simulink model "demodulation"  (R2022b)
settings: Solver=VariableStepAuto  StartTime=0.0  StopTime=1  RelTol=1e-3
libraries: commsynccomp2 x2, dspfdesign x1
settings Model: Creator=Samin  LastModifiedBy=Samin

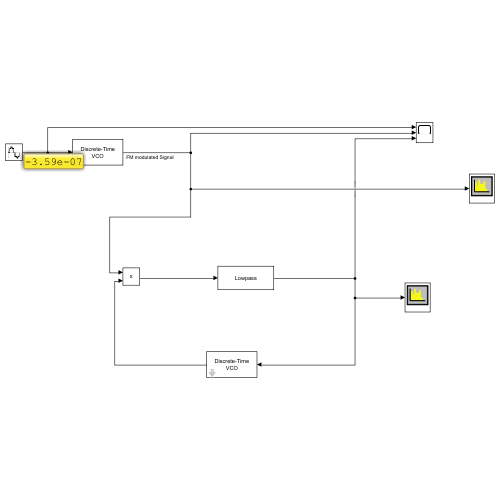
[thumbnail: Simulink's stored preview of the top-level diagram]
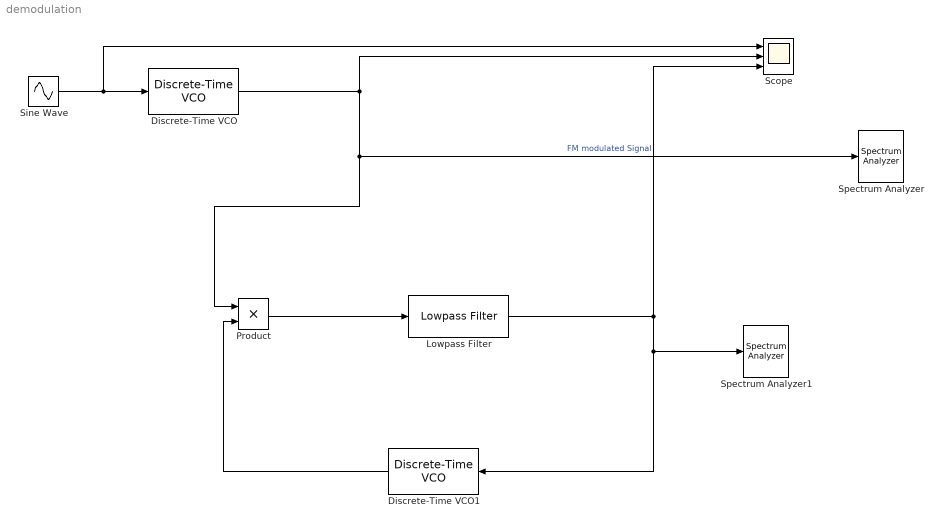
== system demodulation ==
  Discrete-Time VCO : commsynccomp2/Discrete-Time VCO  Ac=1  Fc=10000  Kc=2500  Ph=0  ts=1/2e5
  Discrete-Time VCO1 : commsynccomp2/Discrete-Time VCO  Ac=1  Fc=10000  Kc=100  Ph=0  ts=1/2e5
  Lowpass Filter : dspfdesign/Lowpass Filter  FilterType=FIR  DesignForMinimumOrder=on  FilterOrder=50  PassbandFrequency=2500  StopbandFrequency=3500  PassbandRipple=0.1  StopbandAttenuation=80  InheritSampleRate=off  SampleRate=200e3  SimulateUsing=Interpreted execution  roundingMode=Floor  coeffsDataTypeStr=fixdt(1,16)
  Product : Product  Description=Matrix Multiply
  Scope : Scope  NumInputPorts=3
  Sine Wave : Sin  Frequency=12566.370614  SampleTime=0.00001
  Spectrum Analyzer : SpectrumAnalyzer
  Spectrum Analyzer1 : SpectrumAnalyzer
  wires:
  Discrete-Time VCO1/1 -> Product/2
  Lowpass Filter/1 -> Spectrum Analyzer1/1, Discrete-Time VCO1/1, Scope/3
  Discrete-Time VCO/1 -> Spectrum Analyzer/1, Product/1, Scope/2  "FM modulated Signal"
  Product/1 -> Lowpass Filter/1
  Sine Wave/1 -> Discrete-Time VCO/1, Scope/1
